simulink library "pmm"  (R2021b)
settings: Solver=VariableStepAuto  StartTime=0.0  StopTime=10.0  RelTol=1e-3
undefined symbols (not defined in the file or in its folder): APMM_CoolgFanActCurr_X_pct, APMM_EWP1Curr_X_c, APMM_EWP3Curr_X_c, APMM_LVBattChktime_X_enum, APMM_LVBattChrgtime_X_enum, APMM_LVChrgLv_X_mV, ENUM_ANTITHEFT_ALARM, ENUM_ANTITHEFT_ARM, ENUM_ANTITHEFT_DISARM, ENUM_ANTITHEFT_WAIT, ENUM_CHRGPLUGSTA_NONE, ENUM_CRASHSTATE_NOCRASH, ENUM_DCDCFAULTSTA_ANYFAULTLV1, ENUM_DCDCFAULTSTA_ANYFAULTLV2, ENUM_DRIVETRAIN_AWD, ENUM_DRIVETRAIN_FWD, ENUM_DRIVETRAIN_RWD, ENUM_GEARACTUALPOSN_D, ENUM_GEARACTUALPOSN_N, ENUM_GEARACTUALPOSN_R, ENUM_HVBATTREADYPRE_READY, ENUM_OTACHKSTA_NOREQUEST, ENUM_OTACHKSTA_NOTIMEOUT, ENUM_OTACHKSTA_TIMEOUT, ENUM_PDKEYRAWLULOCK_INLOCK, ENUM_PDKEYRAWLULOCK_INUNLOCK, ENUM_PDKEYRAWPS_INPS, ENUM_PDKEYSTA_LOCK, ENUM_PDKEYSTA_PS, ENUM_PDKEYSTA_UNAVALIABLE, ENUM_PDKEYSTA_UNLOCK, ENUM_POWERSTA_OFF, ENUM_POWERSTA_OFFC, ENUM_POWERSTA_STANDBY, ENUM_PWRREQOTA_REQPOWEROFF, ENUM_PWRREQOTA_REQPOWERSTDBY, ENUM_PWRSTASW_READY, FALSE, KPMM_AllDoorClosedHoldTime_s, KPMM_APSAllowThd_pct, KPMM_BattDownFailtime_s, KPMM_BattUpFailtime_s, KPMM_BattUpResetRty_cnt, KPMM_BattUpResetSW_flg, KPMM_BattUpResetTO_s, KPMM_BattUpRstDlyTO_s, KPMM_BrakeSWHoldTime_s, KPMM_ChrgPlugHoldTime_s, KPMM_DCDCDisableFailtime_s, KPMM_DCDCEnableFailtime_s, KPMM_DCDCVSET_V, KPMM_DCDCVSETLVChrg_V, KPMM_DoorSWHoldTime_s, KPMM_DriverSafetyChkFailtime_s, KPMM_DrivetrainSelect_enum_ovrdflg, KPMM_DrivetrainSelect_enum_ovrdval, KPMM_FDADC12VDetAccu_s, KPMM_FDADC12VDetAccuIntval_s, KPMM_FirstLVCheckHoldT_s, KPMM_FrMCUDischrgVolt_V ... (+54)
libraries: simulink x28, hcu_lib x13
(part 5 of 5)

== stateflow chart pmm/PMM/PMM/RequirementManagementForPowerDown ==
  state RequirementManagementForPowerDown
    (default) -> (junction 2) : {
        |  VPMM_LowSOCWarn_enum = ENUM_LOWSOCWARN_NORMAL;
        |  VPMM_HVSOCWarnTimer_s = 0;
        |  VPMM_SysPwrDownDbns_s = 0;
        | }
    RequirementManagementForPowerDown -> (junction 2)
    (junction 2) -> (junction 3) : {VPMM_PwrDownReq_enum = ENUM_PWRDOWNREQ_NOREQUEST;}
    (junction 3) -> (junction 4) [order 1] : [VPMM_PowerSta_enum == ENUM_POWERSTA_ON || ...
        |  VPMM_PowerSta_enum == ENUM_POWERSTA_OFFA || ...
        |  VPMM_PowerSta_enum == ENUM_POWERSTA_OFFC]
    (junction 4) -> (junction 5) [commented out] : [VINP_IVIPwroffreq_flg]
    (junction 3) -> (junction 7) [order 2]
    (junction 4) -> (junction 11)
    (junction 5) -> (junction 8) [commented out] : {VPMM_PwrDownReq_enum = ENUM_PWRDOWNREQ_USERREQPD;}
    (junction 11) -> (junction 10) [order 1] : [VPMM_PwrStaConstraint_enum == ENUM_PWRCONSTRAINT_NOREQUEST]
    (junction 10) -> (junction 18)
    (junction 11) -> (junction 12) [order 2]
    (junction 12) -> (junction 13) [order 1] : [VINP_HVBattSOC_pct >= KPMM_HVSOCWarnThd_pct]
    (junction 12) -> (junction 107) [order 2]
    (junction 13) -> (junction 14) : {
        |  VPMM_HVSOCWarnTimer_s = 0;
        |  VPMM_LowSOCWarn_enum = ENUM_LOWSOCWARN_NORMAL;
        | }
    (junction 107) -> (junction 14) [order 2] : {VPMM_HVSOCWarnTimer_s += task_time_s;}
    (junction 107) -> (junction 15) [order 1] : [VPMM_HVSOCWarnTimer_s >= KPMM_HVSOCWarnTime_s]
    (junction 15) -> (junction 16) [order 1] : [VINP_HVBattSOC_pct < KPMM_HVSOCWarnThd_pct && ...
        |  VINP_HVBattSOC_pct >= KPMM_HVBattSOCPwrDwnThd_pct]
    (junction 16) -> (junction 17) [commented out] : [VINP_ExtChrgSta_enum == ENUM_EXTCHRGSTS_CHARGING]
    (junction 15) -> (junction 19) [order 2] : {VPMM_LowSOCWarn_enum = ENUM_LOWSOCWARN_HVSOCLOW;}
    (junction 16) -> (junction 20) : {VPMM_LowSOCWarn_enum = ENUM_LOWSOCWARN_HVSOCLOW;}
    (junction 18) -> (junction 121) [order 1] : [VPMM_OTAPwrReqOFFChkSta_enum == ENUM_OTACHKSTA_NOTIMEOUT || ...
        |  VPMM_PwrStaTOSta_enum == ENUM_PWRSTATOSTA_TIMEOUT || ...
        |  VPMM_Sched_ChgTOSta_enum == ENUM_SCHEDCHGTO_TIMEOUT || ...
        |  VPMM_LVSilentChrgSta_enum == ENUM_SILENTCHRGSTA_FAULT || ...
        |  (((VPMM_DetectHVPwrSta_flg && VPMM_PowerSta_enum == ENUM_POWERSTA_ON) || ...
        |    VINP_RePwrReqTbox_enum == ENUM_REPWRREQTBOX_REQPWROFF || ...
        |    VPMM_TCountSta_enum == ENUM_TCOUNTSTA_COUNTINGFINISH) && ...
        |   VPMM_AllDoorClosed_flg && ...
        |   !VINP_SeatSW_flg && ...
        |   !VPMM_BrkPedalPressed_flg)]
    (junction 121) -> (junction 19) [order 1] : [VPMM_SysPwrDownDbns_s >= KPMM_SysPwrDownDbns_s]
    (junction 18) -> (junction 21) [order 2] : {VPMM_SysPwrDownDbns_s = 0;}
    (junction 121) -> (junction 114) [order 2] : {VPMM_SysPwrDownDbns_s += task_time_s;}
    (junction 19) -> (junction 23)
    (junction 21) -> (junction 95) [order 1] : [VPMM_PowerSta_enum == ENUM_POWERSTA_OFFA]
    (junction 95) -> (junction 23) [order 1] : [(VPMM_OffA2OffTimeCnt_s > KPMM_OffA2OffTime_s && ...
        |   !VINP_EvccAplusPwrUpReq_flg) || ...
        |  VINP_HoodSW_flg]
    (junction 21) -> (junction 97) [order 2] : {VPMM_OffA2OffTimeCnt_s = 0;}
    (junction 95) -> (junction 99) [order 2] : {VPMM_OffA2OffTimeCnt_s += task_time_s;}
    (junction 23) -> (junction 25) : {VPMM_PwrDownReq_enum = ENUM_PWRDOWNREQ_SYSREQPD;
        |  VPMM_OffA2OffTimeCnt_s = 0;
        |  VPMM_SysPwrDownDbns_s = 0;}
  data: task_time_s input; KPMM_HVSOCWarnThd_pct input; KPMM_OffA2OffTime_s input; VINP_HVBattSOC_pct input; VPMM_PowerSta_enum input; VPMM_PwrStaConstraint_enum input; VPMM_PwrStaTOSta_enum input; VPMM_TCountSta_enum input; VINP_RePwrReqTbox_enum input; VPMM_LowSOCWarn_enum output; VPMM_PwrDownReq_enum output; VPMM_OffA2OffTimeCnt_s local single; ENUM_LOWSOCWARN_HVSOCLOW parameter; ENUM_LOWSOCWARN_NORMAL parameter; ENUM_POWERSTA_OFFA parameter; ENUM_POWERSTA_OFFC parameter; ENUM_POWERSTA_ON parameter; ENUM_PWRCONSTRAINT_NOREQUEST parameter; ENUM_PWRDOWNREQ_NOREQUEST parameter; ENUM_PWRDOWNREQ_SYSREQPD parameter; ENUM_PWRSTATOSTA_TIMEOUT parameter; ENUM_REPWRREQTBOX_REQPWROFF parameter; ENUM_TCOUNTSTA_COUNTINGFINISH parameter; VPMM_Sched_ChgTOSta_enum input; ENUM_SCHEDCHGTO_TIMEOUT parameter; VPMM_LVSilentChrgSta_enum input; ENUM_SILENTCHRGSTA_FAULT parameter; KPMM_HVSOCWarnTime_s input; VPMM_HVSOCWarnTimer_s local double; VINP_HoodSW_flg input; VPMM_AllDoorClosed_flg input; VPMM_DetectHVPwrSta_flg input; VINP_SeatSW_flg input; KPMM_SysPwrDownDbns_s input; VPMM_SysPwrDownDbns_s local single; VPMM_BrkPedalPressed_flg input; VINP_EvccAplusPwrUpReq_flg input; KPMM_HVBattSOCPwrDwnThd_pct input; VPMM_OTAPwrReqOFFChkSta_enum input uint8; ENUM_OTACHKSTA_NOTIMEOUT parameter
